simulink model "simulazione_001_s"  (R2016b)
settings: Solver=ode4  StartTime=0.0  StopTime=t_sim  FixedStep=step  RelTol=1e-3
values from neighbouring files (symbols this model uses):
  delta_x = -0.5    [simulazione_001_init.m]
  gain = 20 * eye(6)    [simulazione_001_init.m]
  movement_lower_limit = -movement_upper_limit    [simulazione_001_init.m]
  movement_upper_limit = [2*pi; 2*pi; 2*pi; 2*pi; 2*pi; 2*pi]    [simulazione_001_init.m]
  p_init = direct_kinematic(q_init)    [simulazione_001_init.m]
  q_init = [0; 0; 0; 0; 0; 0]    [simulazione_001_init.m]
  t_exe = 2    [simulazione_001_init.m]
  velocity_lower_limit = -velocity_upper_limit    [simulazione_001_init.m]
  velocity_upper_limit = [2*pi/3; 2*pi/3; pi; pi; pi; pi]    [simulazione_001_init.m]
settings Model: Creator=IBM  LastModifiedBy=IBM

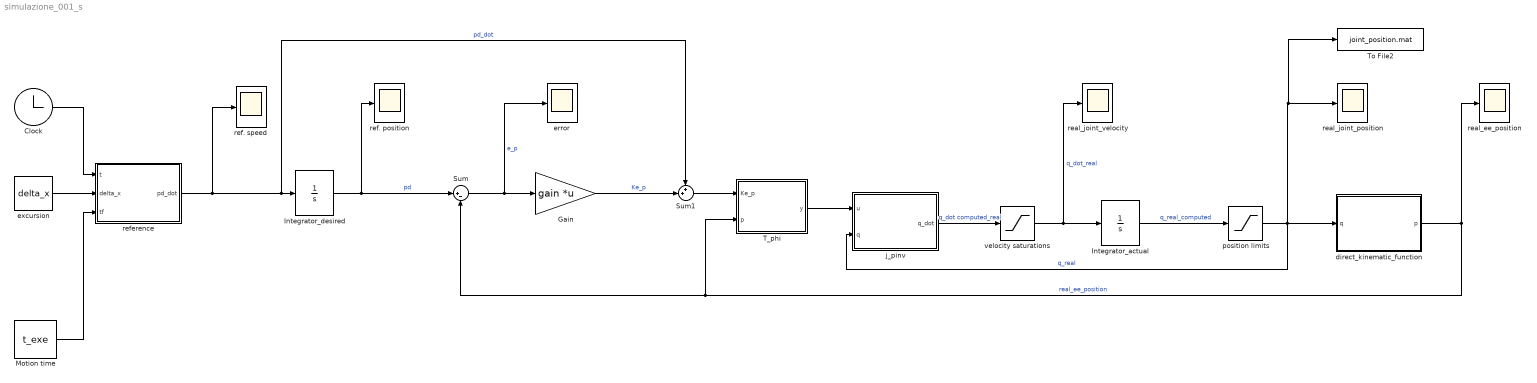
== system simulazione_001_s ==
  Clock : Clock
  Gain : Gain  Gain=gain  Multiplication=Matrix(K*u) (u vector)
  Integrator_actual : Integrator  InitialCondition=q_init
  Integrator_desired : Integrator  InitialCondition=p_init
  Motion time : Constant  Value=t_exe
  Sum : Sum  Inputs=|+-
  Sum1 : Sum  Inputs=++|
  T_phi : MATLAB Function  TreatAsAtomicUnit=on
  To File2 : ToFile  Filename=joint_position.mat  MatrixName=q
  direct_kinematic_function : MATLAB Function  TreatAsAtomicUnit=on
  error : Scope
  excursion : Constant  Value=delta_x
  j_pinv : MATLAB Function  TreatAsAtomicUnit=on
  position limits : Saturate  UpperLimit=movement_upper_limit  LowerLimit=movement_lower_limit
  real_ee_position : Scope
  real_joint_position : Scope
  real_joint_velocity : Scope
  ref. position : Scope
  ref. speed : Scope
  reference : MATLAB Function  TreatAsAtomicUnit=on
  velocity saturations : Saturate  UpperLimit=velocity_upper_limit  LowerLimit=velocity_lower_limit
  wires:
  Clock/1 -> reference/1(t)
  Integrator_desired/1 -> ref. position/1, Sum/1  "pd"
  Motion time/1 -> reference/3(tf)
  Sum/1 -> error/1, Gain/1  "e_p"
  Integrator_actual/1 -> position limits/1  "q_real_computed"
  direct_kinematic_function/1(p) -> real_ee_position/1, T_phi/2(p), Sum/2  "real_ee_position"
  excursion/1 -> reference/2(delta_x)
  reference/1(pd_dot) -> ref. speed/1, Sum1/1, Integrator_desired/1  "pd_dot"
  position limits/1 -> j_pinv/2(q), To File2/1, real_joint_position/1, direct_kinematic_function/1(q)  "q_real"
  velocity saturations/1 -> real_joint_velocity/1, Integrator_actual/1  "q_dot_real"
  j_pinv/1(q_dot) -> velocity saturations/1  "q_dot computed_real"
  T_phi/1(y) -> j_pinv/1(u)
  Gain/1 -> Sum1/2  "Ke_p"
  Sum1/1 -> T_phi/1(Ke_p)

== matlab function simulazione_001_s/j_pinv ==
  data: u input; q_dot output; q input
function q_dot = j_pinv(u, q)
    
    J = geometric_jacobian(q);    
    J_p = pinv(J);
    q_dot = J_p*u;
    
end

== matlab function simulazione_001_s/reference ==
  data: t input; delta_x input; pd_dot output; tf input
function pd_dot = reference(t, delta_x, tf)

    pd_dot = linear_reference(t, delta_x, tf);
    
end

== matlab function simulazione_001_s/direct_kinematic_function ==
  data: q input; p output
function p = dkf(q)

    p = direct_kinematic(q);

== matlab function simulazione_001_s/T_phi ==
  data: Ke_p input; y output; p input
function y = T_phi(Ke_p, p)
        
    t_phi_matrix = [0,  -sin(p(4)),     cos(p(4))*sin(p(5));
                    0,   cos(p(4)),     sin(p(4))*sin(p(5));
                    1,       0,             cos(p(5))];
            
    t_phi_matrix_6x6 = [ eye(3),   zeros(3);
                        zeros(3), t_phi_matrix];
    
    y = t_phi_matrix_6x6 * Ke_p;
end
